simulink model "CommonModeSimulation"  (R2023b)
settings: Solver=FixedStepAuto  StartTime=0.0  StopTime=1/ffund  FixedStep=1e-8  RelTol=1e-3
InitFcn:
  | fsw=1e3;
  | ma=0.60;
  | ffund=100;
settings Model: Creator=enesa  LastModifiedBy=enesa

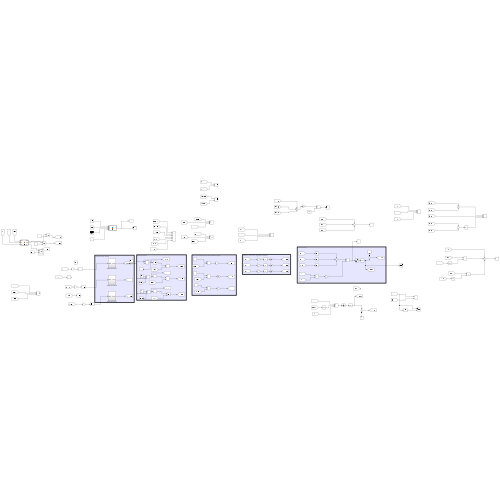
[thumbnail: Simulink's stored preview of the top-level diagram]
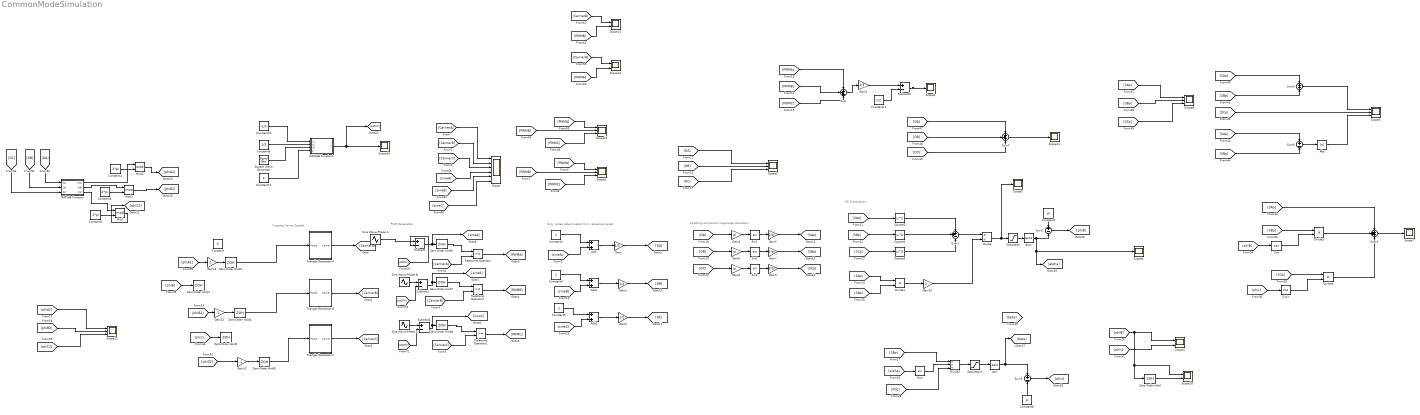
== system CommonModeSimulation ==
  note: Phi B calculation
  note: Switching component magnitude calculation
  note: Duty cycles determination from reference signals
  note: PWM Generation
  note: Creating Carrier Signals
  Abs : Abs  SaturateOnIntegerOverflow=off
  Acos : Trigonometry  Operator=acos
  Add : Sum
  Add1 : Sum
  Add2 : Sum
  Asin : Trigonometry  Operator=asin
  Constant : Constant  Value=0
  Constant1 : Constant  Value=2*pi
  Constant10 : Constant  Value=-1/3
  Constant11 : Constant  Value=4
  Constant12 : Constant  Value=1/2
  Constant2 : Constant  Value=2*pi
  Constant3 : Constant
  Constant4 : Constant
  Constant5 : Constant
  Constant6 : Constant  Value=1/3
  Constant7 : Constant  Value=pi
  Constant8 : Constant  Value=pi
  Constant9 : Constant  Value=2*pi
  Cos : Trigonometry  Operator=cos
  Cos1 : Trigonometry  Operator=cos
  Divide : Product  Inputs=*/
  Divide1 : Product  Inputs=**
  Divide2 : Product  Inputs=**/
  Divide3 : Product  Inputs=**
  Divide4 : Product  Inputs=**
  Gain : Gain  Gain=1/2
  Gain1 : Gain  Gain=1/2
  Gain10 : Gain  Gain=2
  Gain11 : Gain  Gain=-1
  Gain12 : Gain  Gain=-1
  Gain13 : Gain  Gain=-1
  Gain2 : Gain  Gain=1/2
  Gain3 : Gain  Gain=1/3
  Gain4 : Gain  Gain=pi
  Gain5 : Gain  Gain=2/pi
  Gain6 : Gain  Gain=pi
  Gain7 : Gain  Gain=2/pi
  Gain8 : Gain  Gain=pi
  Gain9 : Gain  Gain=2/pi
  MATLAB Function : MATLAB Function  TreatAsAtomicUnit=on
  MATLAB Function1 : MATLAB Function  TreatAsAtomicUnit=on
  Mod : Math  Operator=mod
  Mod1 : Math  Operator=mod
  Mod2 : Math  Operator=mod
  Relational Operator : RelationalOperator  OutDataTypeStr=boolean  RndMeth=Simplest  InputSameDT=off
  Relational Operator1 : RelationalOperator  OutDataTypeStr=boolean  RndMeth=Simplest  InputSameDT=off
  Relational Operator2 : RelationalOperator  OutDataTypeStr=boolean  RndMeth=Simplest  InputSameDT=off
  Saturation : Saturate  UpperLimit=1  LowerLimit=-1
  Saturation1 : Saturate  UpperLimit=1  LowerLimit=-1
  Scope : Scope  NumInputPorts=6
  Scope{1,3,8..9,12,15} (6 alike) : Scope  NumInputPorts=3
  Scope{4,10,13..14} (4 alike) : Scope  NumInputPorts=2
  Scope{2,5..7,11,16} (6 alike) : Scope
  Sin{1..4} (4 alike) : Trigonometry
  Sine Wave-Phase A : Sin  Amplitude=ma  Frequency=2*pi*ffund  SampleTime=0
  Sine Wave-Phase B : Sin  Amplitude=ma  Frequency=2*pi*ffund  Phase=2*pi/3  SampleTime=0
  Sine Wave-Phase C : Sin  Amplitude=ma  Frequency=2*pi*ffund  Phase=-2*pi/3  SampleTime=0
  Square Wave Generator : SignalGenerator  WaveForm=square  Amplitude=1/3  Frequency=2*pi*ffund*3  Units=rad/sec
  Square1 : Math  Operator=square
  Square2 : Math  Operator=square
  Square3 : Math  Operator=square
  Subtract{,1..3} (4 alike) : Sum  Inputs=+-
  Sum : Sum  Inputs=+++
  Sum1 : Sum  Inputs=++-
  Sum2 : Sum  Inputs=+-
  Sum3 : Sum  Inputs=+-
  Sum4 : Sum  Inputs=+++
  Sum5 : Sum
  Sum6 : Sum  Inputs=+-
  Sum7 : Sum  Inputs=+++
  Triangle Generator-A : Subsystem
  Triangle Generator-B : Subsystem
  Triangle Generator-C : Subsystem
  Zero-Order Hold{,1..8} (9 alike) : ZeroOrderHold  SampleTime=1/fsw
  wires:
  [CarrierA] -> Scope/1
  [CarrierB] -> Scope/2
  [CarrierC] -> Scope/3
  [PWMA] -> Scope1/1
  [PWMB] -> Scope1/2
  [PWMC] -> Scope1/3
  [PWMA] -> Sum/1
  [PWMB] -> Sum/2
  [PWMC] -> Sum/3
  Sum/1 -> Gain3/1
  [DA] -> Scope3/1
  [DB] -> Scope3/2
  [DC] -> Scope3/3
  Triangle Generator-C/1(Carrier) -> [CarrierC]
  Triangle Generator-B/1(Carrier) -> [CarrierB]
  Triangle Generator-A/1(Carrier) -> [CarrierA]
  [CarrierB] -> Relational Operator1/2
  Relational Operator1/1 -> [PWMB]
  Relational Operator/1 -> [PWMA]
  Relational Operator2/1 -> [PWMC]
  [CarrierC] -> Relational Operator2/2
  Sine Wave-Phase A/1 -> Subtract/1
  [CarrierA] -> Relational Operator/2
  Sine Wave-Phase B/1 -> Subtract1/1
  [sineC] -> Add2/2
  Constant4/1 -> Add1/1
  Constant3/1 -> Add/1
  Add2/1 -> Gain2/1
  Gain/1 -> [DA]
  Gain2/1 -> [DC]
  Add1/1 -> Gain1/1
  [sineB] -> Add1/2
  Constant5/1 -> Add2/1
  [sineA] -> Add/2
  Gain1/1 -> [DB]
  Add/1 -> Gain/1
  [DA] -> Gain4/1
  Sin1/1 -> Gain5/1
  Gain4/1 -> Sin1/1
  [DB] -> Gain6/1
  Gain7/1 -> [SBp]
  Sin3/1 -> Gain9/1
  Gain6/1 -> Sin2/1
  Gain8/1 -> Sin3/1
  [DC] -> Gain8/1
  Gain5/1 -> [SAp]
  Gain9/1 -> [SCp]
  Sin2/1 -> Gain7/1
  [SCp] -> Square3/1
  Acos/1 -> Sum2/2, Scope6/1, [alpha]
  Gain10/1 -> Divide/2
  Square3/1 -> Sum1/3
  [SAp] -> Divide1/1
  Sum1/1 -> Divide/1
  [SBp] -> Square1/1
  [SBp] -> Divide1/2
  Constant7/1 -> Sum2/1
  Divide/1 -> Scope5/1, Saturation/1
  Square2/1 -> Sum1/1
  [SAp] -> Square2/1
  Sum2/1 -> [phiB]
  Square1/1 -> Sum1/2
  Divide1/1 -> Gain10/1
  [alpha] -> Sin4/1
  [SBp] -> Divide2/1
  Sin4/1 -> Divide2/2
  [SCp] -> Divide2/3
  Divide2/1 -> Saturation1/1
  Asin/1 -> Sum3/1, [beta]
  Constant8/1 -> Sum3/2
  Sum3/1 -> [phic]
  [phiB] -> Scope10/1, Zero-Order Hold/1, Scope4/1
  [phic] -> Scope4/2
  [SBp] -> Divide3/1
  [phiB] -> Cos/1
  Cos/1 -> Divide3/2
  [phic] -> Cos1/1
  Cos1/1 -> Divide4/2
  [SCp] -> Divide4/1
  [SAp] -> Sum4/1
  Divide3/1 -> Sum4/2
  Divide4/1 -> Sum4/3
  Sum4/1 -> Scope7/1
  [SAp] -> Scope8/1
  [SBp] -> Scope8/2
  [SCp] -> Scope8/3
  [SAp] -> Sum5/1
  [SBp] -> Sum5/2
  Sum5/1 -> Scope9/1
  [SCp] -> Scope9/2
  [SAp] -> Sum6/1
  [SBp] -> Sum6/2
  Sum6/1 -> Abs/1
  Abs/1 -> Scope9/3
  Saturation/1 -> Acos/1
  Saturation1/1 -> Asin/1
  Zero-Order Hold/1 -> Scope10/2
  [DA] -> Sum7/1
  [DC] -> Sum7/3
  [DB] -> Sum7/2
  Sum7/1 -> Scope11/1
  [phiB2] -> Scope12/2
  [phiC2] -> Scope12/3
  [DA] -> MATLAB Function/1(DA)
  [DB] -> MATLAB Function/2(DB)
  [DC] -> MATLAB Function/3(DC)
  [phiA2] -> Scope12/1
  [phic] -> Zero-Order Hold2/1
  [phiB] -> Zero-Order Hold1/1
  [CarrierA] -> Scope13/1
  [PWMA] -> Scope13/2
  [CarrierA] -> Scope14/1
  [PWMB] -> Scope14/2
  [phiC2] -> Gain11/1
  [phiB2] -> Gain12/1
  [phiA2] -> Gain13/1
  Constant1/1 -> Mod/2
  Constant2/1 -> Mod1/2
  Constant9/1 -> Mod2/2
  Mod2/1 -> [phiB2]
  Mod/1 -> [phiC2]
  Mod1/1 -> [phiA2]
  MATLAB Function/1(phA) -> Mod1/1
  MATLAB Function/2(phB) -> Mod2/1
  MATLAB Function/3(phC) -> Mod/1
  Gain13/1 -> Zero-Order Hold3/1
  Gain12/1 -> Zero-Order Hold4/1
  Gain11/1 -> Zero-Order Hold5/1
  Zero-Order Hold3/1 -> Triangle Generator-A/1(Phase)
  Zero-Order Hold4/1 -> Triangle Generator-B/1(Phase)
  Zero-Order Hold5/1 -> Triangle Generator-C/1(Phase)
  Zero-Order Hold6/1 -> Relational Operator/1
  Zero-Order Hold7/1 -> Relational Operator1/1
  Zero-Order Hold8/1 -> Relational Operator2/1
  [PWMB] -> Scope15/2
  [PWMC] -> Scope15/3
  [PWMA] -> Scope15/1
  [sineA] -> Scope/4
  [sineB] -> Scope/5
  [sineC] -> Scope/6
  Subtract/1 -> [sineA], Zero-Order Hold6/1
  [sqCMV] -> Subtract/2
  Subtract1/1 -> [sineB], Zero-Order Hold7/1
  [sqCMV] -> Subtract1/2
  Sine Wave-Phase C/1 -> Subtract2/1
  Subtract2/1 -> [sineC], Zero-Order Hold8/1
  [sqCMV] -> Subtract2/2
  Constant6/1 -> MATLAB Function1/2(u2)
  Square Wave Generator/1 -> MATLAB Function1/3(u3)
  MATLAB Function1/1(y) -> [sqCMV], Scope16/1
  Constant10/1 -> MATLAB Function1/1(u1)
  Constant11/1 -> MATLAB Function1/4(d)
  Gain3/1 -> Subtract3/1
  Subtract3/1 -> Scope2/1
  Constant12/1 -> Subtract3/2

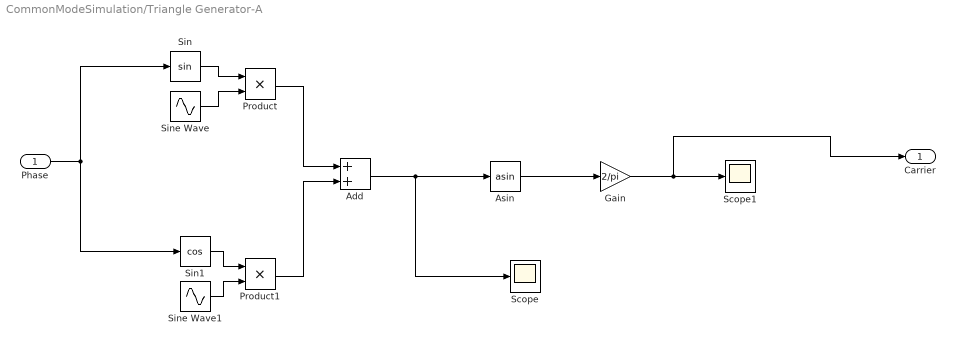
== system CommonModeSimulation/Triangle Generator-A ==
  Phase : Inport
  Add : Sum
  Asin : Trigonometry  Operator=asin
  Gain : Gain  Gain=2/pi
  Product : Product
  Product1 : Product
  Scope : Scope
  Scope1 : Scope
  Sin : Trigonometry
  Sin1 : Trigonometry  Operator=cos
  Sine Wave : Sin  Frequency=2*pi*fsw  SampleTime=0
  Sine Wave1 : Sin  Frequency=2*pi*fsw  Phase=-pi/2  SampleTime=0
  Carrier : Outport
  wires:
  Sin/1 -> Product/1
  Sine Wave/1 -> Product/2
  Phase/1 -> Sin1/1, Sin/1
  Product/1 -> Add/1
  Asin/1 -> Gain/1
  Gain/1 -> Carrier/1, Scope1/1
  Sine Wave1/1 -> Product1/2
  Product1/1 -> Add/2
  Add/1 -> Asin/1, Scope/1
  Sin1/1 -> Product1/1

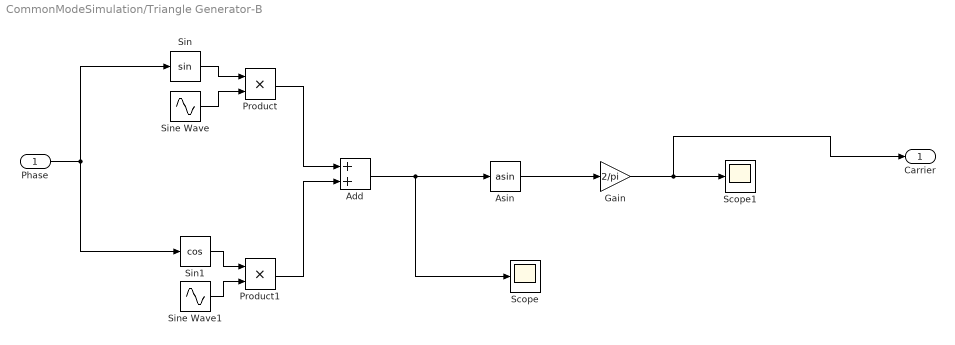
== system CommonModeSimulation/Triangle Generator-B ==
  Phase : Inport
  Add : Sum
  Asin : Trigonometry  Operator=asin
  Gain : Gain  Gain=2/pi
  Product : Product
  Product1 : Product
  Scope : Scope
  Scope1 : Scope
  Sin : Trigonometry
  Sin1 : Trigonometry  Operator=cos
  Sine Wave : Sin  Frequency=2*pi*fsw  SampleTime=0
  Sine Wave1 : Sin  Frequency=2*pi*fsw  Phase=-pi/2  SampleTime=0
  Carrier : Outport
  wires:
  Sin/1 -> Product/1
  Sine Wave/1 -> Product/2
  Phase/1 -> Sin1/1, Sin/1
  Product/1 -> Add/1
  Asin/1 -> Gain/1
  Gain/1 -> Carrier/1, Scope1/1
  Sine Wave1/1 -> Product1/2
  Product1/1 -> Add/2
  Add/1 -> Asin/1, Scope/1
  Sin1/1 -> Product1/1

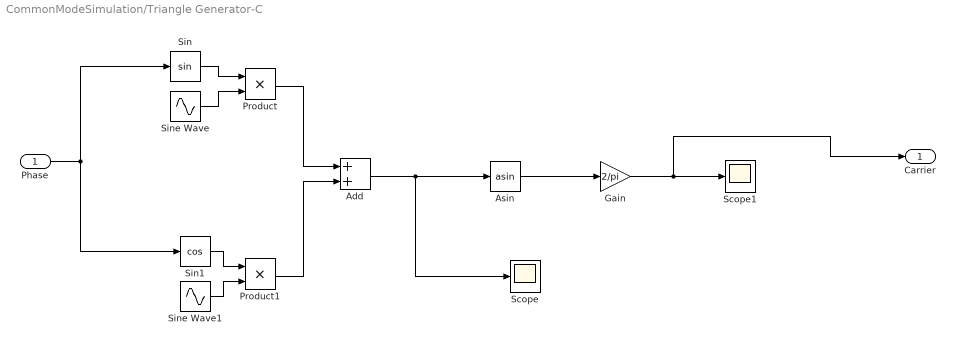
== system CommonModeSimulation/Triangle Generator-C ==
  Phase : Inport
  Add : Sum
  Asin : Trigonometry  Operator=asin
  Gain : Gain  Gain=2/pi
  Product : Product
  Product1 : Product
  Scope : Scope
  Scope1 : Scope
  Sin : Trigonometry
  Sin1 : Trigonometry  Operator=cos
  Sine Wave : Sin  Frequency=2*pi*fsw  SampleTime=0
  Sine Wave1 : Sin  Frequency=2*pi*fsw  Phase=-pi/2  SampleTime=0
  Carrier : Outport
  wires:
  Sin/1 -> Product/1
  Sine Wave/1 -> Product/2
  Phase/1 -> Sin1/1, Sin/1
  Product/1 -> Add/1
  Asin/1 -> Gain/1
  Gain/1 -> Carrier/1, Scope1/1
  Sine Wave1/1 -> Product1/2
  Product1/1 -> Add/2
  Add/1 -> Asin/1, Scope/1
  Sin1/1 -> Product1/1

== matlab function CommonModeSimulation/MATLAB Function1 ==
  data: u1 input; y output; u2 input; u3 input; d input
function y = fcn(u1,u2,u3,d)

if d==1
    y = u1;
elseif  d==2
    y = u2;
elseif  d==3
    y = u3;
else
    y = 0;
end

== matlab function CommonModeSimulation/MATLAB Function ==
  data: DA input; phA output; DB input; DC input; phB output; phC output
function [phA, phB,phC] = fcn(DA,DB,DC)
phA=0;
phB=((DA+DB)/2)*2*pi;
phC= (((DA+DC)/2)+DB)*2*pi;
end
